simulink model "swing_up_part2A"  (R2022a)
settings: Solver=ode5  StartTime=0.0  StopTime=100  FixedStep=0.001  RelTol=1e-3  EnableMultiTasking=on
undefined symbols (not defined in the file): HIL
libraries: simulink x7, quarc_library x4, simulink_extras x1
settings Model: Creator=edrozari  LastModifiedBy=afernan8
settings SolverCC: PositivePriorityOrder=on  AutoInsertRateTranBlk=on
settings RTWCC: Description=QUARC Win64 Target Using Toolchain  SystemTargetFile=quarc_win64.tlc  Toolchain=QUARC win64 | nmake (64-bit Windows)  BuildConfiguration=Faster Runs
settings STFCustomTargetCC: TargetLangStandard=C99 (ISO)  ConcurrentExecutionCompliant=on  UseToolchainInfoCompliant=on  SystemTargetFile=quarc_win64.tlc
settings GRTTargetCC: ParMdlRefBuildCompliant=off  CompOptLevelCompliant=off  CombineOutputUpdateFcns=off  MatFileLogging=off  CPPClassGenCompliant=off  GRTInterface=on  ExtMode=on  ExtModeMexFile=quarc_comm

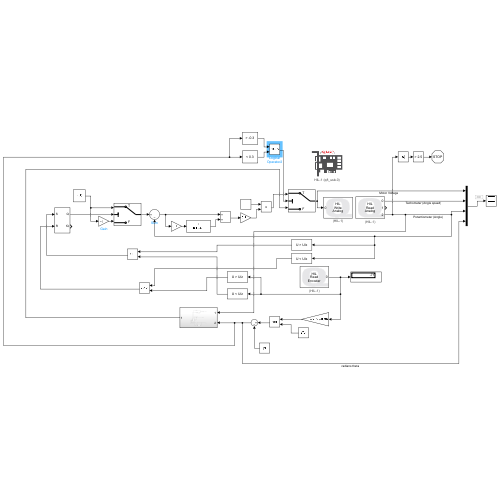
[thumbnail: Simulink's stored preview of the top-level diagram]
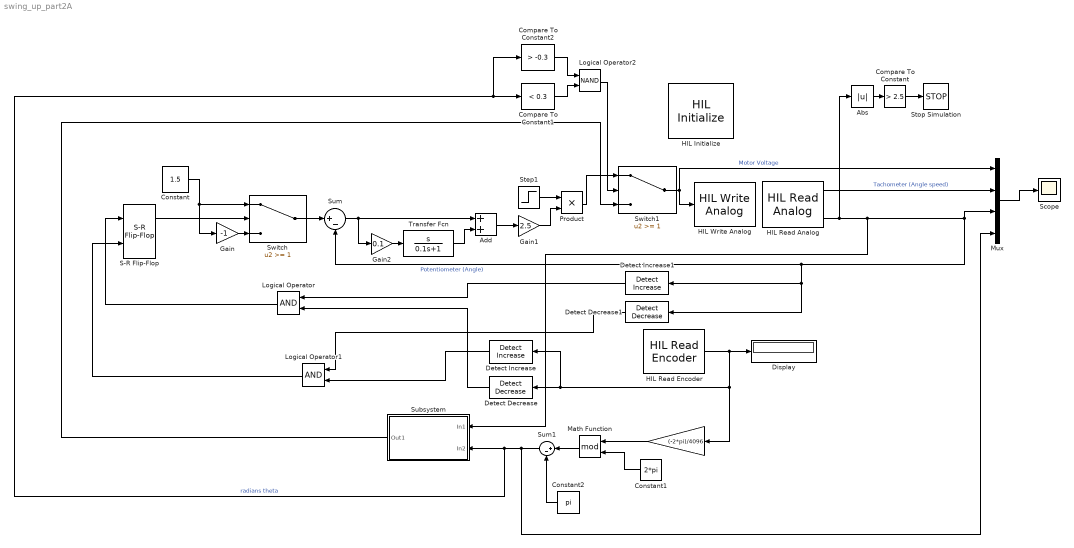
== system swing_up_part2A ==
  "  " : Gain  Gain=(-2*pi)/4096
  Abs : Abs  SaturateOnIntegerOverflow=off
  Add : Sum
  Compare To Constant : simulink/Logic and Bit Operations/Compare To Constant  relop=>  const=2.5  OutDataTypeStr=boolean
  Compare To Constant1 : simulink/Logic and Bit Operations/Compare To Constant  relop=<  const=0.3  OutDataTypeStr=boolean
  Compare To Constant2 : simulink/Logic and Bit Operations/Compare To Constant  relop=>  const=-0.3  OutDataTypeStr=boolean
  Constant : Constant  Value=1.5
  Constant1 : Constant  Value=2*pi
  Constant2 : Constant  Value=pi
  Detect Decrease : simulink/Logic and Bit Operations/Detect Decrease  vinit=0.0  OutDataTypeStr=boolean
  Detect Decrease1 : simulink/Logic and Bit Operations/Detect Decrease  vinit=0.0  OutDataTypeStr=boolean
  Detect Increase : simulink/Logic and Bit Operations/Detect Increase  vinit=0.0  OutDataTypeStr=boolean
  Detect Increase1 : simulink/Logic and Bit Operations/Detect Increase  vinit=0.0  OutDataTypeStr=boolean
  Display : Display
  Gain : Gain  Gain=-1
  Gain1 : Gain  Gain=2.5
  Gain2 : Gain  Gain=0.1
  HIL Initialize : quarc_library/Data Acquisition/Generic/Configuration/HIL Initialize  object_name=HIL-1  board_type=q8_usb  board_number=0  board_options=update_rate=normal;decimation=1  exclusive=off  active=on  hardware_clocks=[0:2]  clock_modes=[]  initial_clock_frequencies=[]  set_clock_params_at_start=off  set_clock_params_at_switch_in=off  set_clock_frequencies_at_start=off  set_clock_frequencies_at_switch_in=off  analog_input_channels=[0:7]  analog_input_configurations=[]  analog_input_maximums=10  analog_input_minimums=-10  set_analog_input_params_at_start=on  set_analog_input_params_at_switch_in=off  analog_output_channels=[0:7]  analog_output_maximums=10  analog_output_minimums=-10  initial_analog_outputs=[0]  final_analog_outputs=[0]  watchdog_analog_outputs=0  set_analog_output_params_at_start=on  set_analog_output_params_at_switch_in=off  set_analog_outputs_at_start=on  set_analog_outputs_at_switch_in=off  set_analog_outputs_at_terminate=on  set_analog_outputs_at_switch_out=off  set_analog_outputs_on_watchdog=off  digital_input_channels=[]  digital_output_channels=[]  digital_output_configuration=[]  initial_digital_outputs=[1]  final_digital_outputs=[1]  watchdog_digital_outputs=[1]  set_digital_output_params_at_start=off  set_digital_output_params_at_switch_in=off  set_digital_outputs_at_start=on  set_digital_outputs_at_switch_in=off  set_digital_outputs_at_terminate=on  set_digital_outputs_at_switch_out=off  set_digital_outputs_on_watchdog=off  encoder_channels=[0:7]  quadrature=[4]  encoder_filter_frequency=[]  initial_encoder_counts=[0]  set_encoder_params_at_start=on  set_encoder_params_at_switch_in=off  set_encoder_counts_at_start=on  set_encoder_counts_at_switch_in=off  pwm_channels=[0:7]  pwm_modes=0  pwm_frequency=99.532799999999995e6/4095  pwm_configuration=[0]  pwm_alignment=[0]  pwm_polarity=[1]  pwm_leading_deadband=[0]  pwm_trailing_deadband=[0]  initial_pwm_outputs=[0]  final_pwm_outputs=[0]  watchdog_pwm_outputs=[0]  set_pwm_params_at_start=on  set_pwm_params_at_switch_in=off  set_pwm_outputs_at_start=on  set_pwm_outputs_at_switch_in=off  set_pwm_outputs_at_terminate=on  set_pwm_outputs_at_switch_out=off  set_pwm_outputs_on_watchdog=off  other_output_channels=[]  initial_other_outputs=[]  final_other_outputs=[]  watchdog_other_outputs=[]  set_other_outputs_at_start=off  set_other_outputs_at_switch_in=off  set_other_outputs_at_terminate=off  set_other_outputs_at_switch_out=off  set_other_outputs_on_watchdog=off
  HIL Read Analog : quarc_library/Data Acquisition/Generic/Immediate I//O/HIL Read Analog  object_name=HIL-1  channels=[0:2]  sample_time=qc_get_step_size  active=on  vector_output=off
  HIL Read Encoder : quarc_library/Data Acquisition/Generic/Immediate I//O/HIL Read Encoder  object_name=HIL-1  channels=0  sample_time=qc_get_step_size  active=on  vector_output=off  data_type_mode=Inherit via back propagation  data_type=double
  HIL Write Analog : quarc_library/Data Acquisition/Generic/Immediate I//O/HIL Write Analog  object_name=HIL-1  channels=[0]  sample_time=-1  active=off  vector_input=off
  Logical Operator : Logic  AllPortsSameDT=off  OutDataTypeStr=boolean
  Logical Operator1 : Logic  AllPortsSameDT=off  OutDataTypeStr=boolean
  Logical Operator2 : Logic  Operator=NAND  AllPortsSameDT=off  OutDataTypeStr=boolean
  Math Function : Math  Operator=mod
  Mux : Mux
  Product : Product
  S-R Flip-Flop : simulink_extras/Flip Flops/S-R Flip-Flop  initial_condition=0
  Scope : Scope
  Step1 : Step  Time=28  Before=1  After=0  SampleTime=0
  Stop Simulation : Stop
  Subsystem : Subsystem
  Sum : Sum  Inputs=|+-
  Sum1 : Sum  Inputs=|+-
  Switch : Switch  Threshold=1  SaturateOnIntegerOverflow=off  InputSameDT=off
  Switch1 : Switch  Threshold=1  SaturateOnIntegerOverflow=off  InputSameDT=off
  Transfer Fcn : TransferFcn  Numerator=[1 0]  Denominator=[0.1 1]
  wires:
  Mux/1 -> Scope/1
  HIL Read Analog/1 -> Mux/2  "Tachometer (Angle speed)"
  HIL Read Analog/3 -> Subsystem/1(In1), Mux/3, Detect Decrease1/1, Detect Increase1/1, Sum/2, Abs/1  "Potentiometer (Angle)"
  Abs/1 -> Compare To Constant/1
  Compare To Constant/1 -> Stop Simulation/1
  Step1/1 -> Product/1
  Constant/1 -> Switch/1, Gain/1
  HIL Read Encoder/1 -> Display/1, Detect Increase/1, Detect Decrease/1, "  "/1
  Gain/1 -> Switch/3
  Switch/1 -> Sum/1
  Sum/1 -> Add/1, Gain2/1
  Gain2/1 -> Transfer Fcn/1
  Transfer Fcn/1 -> Add/2
  Add/1 -> Gain1/1
  Gain1/1 -> Product/2
  Detect Decrease/1 -> Logical Operator/2
  Detect Increase1/1 -> Logical Operator/1
  Detect Increase/1 -> Logical Operator1/2
  Detect Decrease1/1 -> Logical Operator1/1
  Logical Operator/1 -> S-R Flip-Flop/1
  Logical Operator1/1 -> S-R Flip-Flop/2
  S-R Flip-Flop/1 -> Switch/2
  "  "/1 -> Math Function/1
  Constant1/1 -> Math Function/2
  Math Function/1 -> Sum1/1
  Constant2/1 -> Sum1/2
  Switch1/1 -> HIL Write Analog/1, Mux/1  "Motor Voltage"
  Subsystem/1(Out1) -> Switch1/3
  Product/1 -> Switch1/1
  Sum1/1 -> Mux/4, Compare To Constant2/1, Compare To Constant1/1, Subsystem/2(In2)  "radians theta"
  Compare To Constant2/1 -> Logical Operator2/1
  Compare To Constant1/1 -> Logical Operator2/2
  Logical Operator2/1 -> Switch1/2

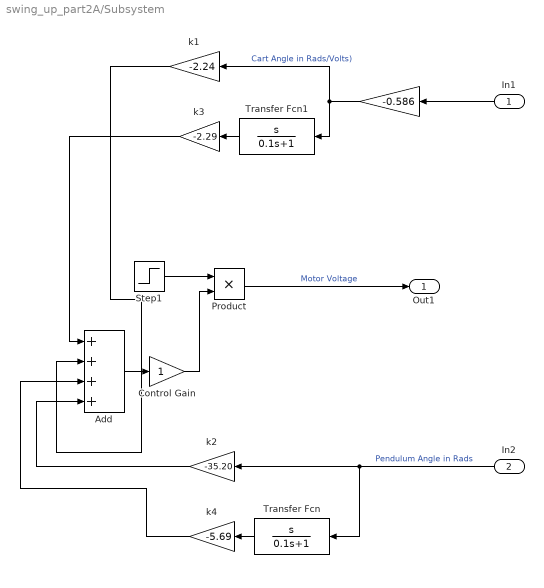
== system swing_up_part2A/Subsystem ==
  In1 : Inport
  In2 : Inport  Port=2
  " " : Gain  Gain=-0.586
  Add : Sum  Inputs=++++
  Control Gain : Gain
  Product : Product
  Step1 : Step  Time=29  Before=1  After=0  SampleTime=0
  Transfer Fcn : TransferFcn  Numerator=[1 0]  Denominator=[0.1 1]
  Transfer Fcn1 : TransferFcn  Numerator=[ 1 0]  Denominator=[0.1 1]
  k1 : Gain  Gain=-2.24
  k2 : Gain  Gain=-35.20
  k3 : Gain  Gain=-2.29
  k4 : Gain  Gain=-5.69
  Out1 : Outport
  wires:
  Step1/1 -> Product/1
  k2/1 -> Add/4
  " "/1 -> k1/1, Transfer Fcn1/1  "Cart Angle in Rads/Volts)"
  Transfer Fcn1/1 -> k3/1
  k3/1 -> Add/1
  Transfer Fcn/1 -> k4/1
  Add/1 -> Control Gain/1
  Control Gain/1 -> Product/2
  In2/1 -> Transfer Fcn/1, k2/1  "Pendulum Angle in Rads"
  k4/1 -> Add/3
  k1/1 -> Add/2
  In1/1 -> " "/1
  Product/1 -> Out1/1  "Motor Voltage"
